simulink model "current_commutated_chopper"  (Simulink 7.5)
settings: Solver=ode45  StartTime=0.0  StopTime=.1  RelTol=1e-3
libraries: powerlib x13
settings Model: Creator=Smrit  LastModifiedBy=Sambhav
settings OptimizationCC: InitFltsAndDblsToZero=on
settings DebuggingCC: SaveWithParameterizedLinksMsg=none  StrictBusMsg=Warning

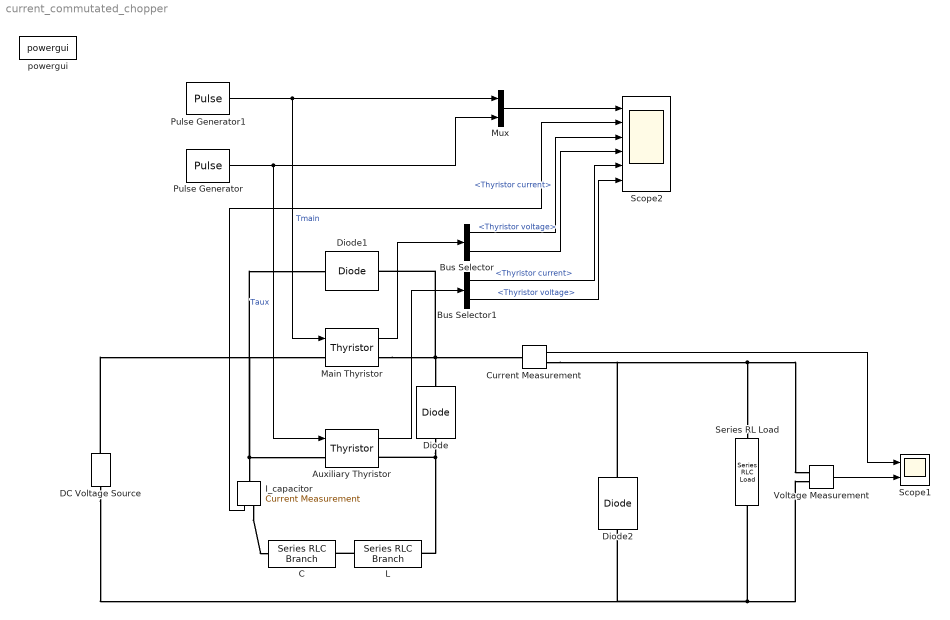
== system current_commutated_chopper ==
  Auxiliary Thyristor : powerlib/Power Electronics/Thyristor  DialogController=POWERSYS.PowerSysDialog  SystemSampleTime=-1  Ron=0.001  Lon=0  Vf=0.8  IC=0  Rs=500  Cs=250e-9  Measurements=on
  Bus Selector : BusSelector  OutputSignals=Thyristor current,Thyristor voltage
  Bus Selector1 : BusSelector  OutputSignals=Thyristor current,Thyristor voltage
  C : powerlib/Elements/Series RLC Branch  DialogController=POWERSYS.PowerSysDialog  PhysicalDomain=powersysdomain  SubClassName=unknown  LeftPortType=p1  RightPortType=p1  LConnTagsString=__new0  RConnTagsString=__new0  BranchType=C  Resistance=1  Inductance=1e-3  SetiL0=off  InitialCurrent=0  Capacitance=1e-6  Setx0=on  InitialVoltage=230  Measurements=None
  Current Measurement : powerlib/Measurements/Current Measurement  DialogController=POWERSYS.PowerSysDialog  SystemSampleTime=-1  PhasorSimulation=off  OutputType=Complex  PSBequivalent=0
  DC Voltage Source : powerlib/Electrical Sources/DC Voltage Source  DialogController=POWERSYS.PowerSysDialog  SystemSampleTime=-1  Amplitude=230  Measurements=None
  Diode : powerlib/Power Electronics/Diode  DialogController=POWERSYS.PowerSysDialog  SystemSampleTime=-1  Ron=0.001  Lon=0  Vf=0.8  IC=0  UseSnubber=off  Rs=500  Cs=250e-9  Measurements=off
  Diode1 : powerlib/Power Electronics/Diode  DialogController=POWERSYS.PowerSysDialog  SystemSampleTime=-1  Ron=0.001  Lon=0  Vf=0.8  IC=0  UseSnubber=off  Rs=500  Cs=250e-9  Measurements=off
  Diode2 : powerlib/Power Electronics/Diode  DialogController=POWERSYS.PowerSysDialog  SystemSampleTime=-1  Ron=0.001  Lon=0  Vf=0.8  IC=0  UseSnubber=off  Rs=500  Cs=250e-9  Measurements=off
  I_capacitor : powerlib/Measurements/Current Measurement  DialogController=POWERSYS.PowerSysDialog  SystemSampleTime=-1  PhasorSimulation=off  OutputType=Complex  PSBequivalent=0
  L : powerlib/Elements/Series RLC Branch  DialogController=POWERSYS.PowerSysDialog  PhysicalDomain=powersysdomain  SubClassName=unknown  LeftPortType=p1  RightPortType=p1  LConnTagsString=__new0  RConnTagsString=__new0  BranchType=L  Resistance=1  Inductance=1e-3  SetiL0=off  InitialCurrent=0  Capacitance=1e-6  Setx0=off  InitialVoltage=0  Measurements=None
  Main Thyristor : powerlib/Power Electronics/Thyristor  DialogController=POWERSYS.PowerSysDialog  SystemSampleTime=-1  Ron=0.001  Lon=0  Vf=0.8  IC=0  Rs=500  Cs=250e-9  Measurements=on
  Mux : Mux  Inputs=2
  Pulse Generator : DiscretePulseGenerator  PulseType=Time based  Amplitude=1  Period=20e-3  PulseWidth=.5  PhaseDelay=10e-3  SampleTime=1
  Pulse Generator1 : DiscretePulseGenerator  PulseType=Time based  Amplitude=1  Period=20e-3  PulseWidth=.5  PhaseDelay=5e-3  SampleTime=1
  Scope1 : Scope  NumInputPorts=2
      settings: YMin=-0.5~-0.2  YMax=3.5~300
  Scope2 : Scope  NumInputPorts=6
      settings: TimeRange=0.01606557841592294  YMin=0~-7~0~-10~0~-10  YMax=1.25~7~4~300~10~300  SaveName=ScopeData2
  Series RL Load : powerlib/Elements/Series RLC Load  DialogController=POWERSYS.PowerSysDialog  PhysicalDomain=powersysdomain  SubClassName=unknown  LeftPortType=p1  RightPortType=p1  LConnTagsString=a  RConnTagsString=__new0  NominalVoltage=1000  NominalFrequency=50  ActivePower=10e3  InductivePower=100  CapacitivePower=0  Setx0=off  InitialVoltage=0  SetiL0=off  InitialCurrent=0  Measurements=None
  Voltage Measurement : powerlib/Measurements/Voltage Measurement  DialogController=POWERSYS.PowerSysDialog  SystemSampleTime=-1  PhasorSimulation=off  OutputType=Complex  PSBequivalent=0
  powergui : powerlib/powergui  SystemSampleTime=-1  SimulationMode=Continuous  SampleTime=50e-6  frequency=60  SPID=off  DisableSnubberDevices=off  DisableRonSwitches=off  DisableVfSwitches=off  SwTol=0  Interpol=off  frequencyindice=0  echomessages=off  HookPort=off  DisplayEquations=off  FunctionMessages=off  EnableUseOfTLC=off  x0status=blocks  RestoreLinks=warning  ResistiveCurrentMeasurement=off  Frange=[0:2:500]  Ylog=off  Xlog=on  ShowGrid=off  save=off  variable=ZData  ZoomFFT=on  StartTime=0.0  cycles=1  DisplayStyle=1  fundamental=60  FreqAxis=off  MaxFrequency=1000  frequencyindicesteady=1  RmsSteady=1  display=off  Ts=0  methode=off
  wires:
  Pulse Generator1/1 -> Main Thyristor/1, Mux/1  "Tmain"
  Pulse Generator/1 -> Auxiliary Thyristor/1, Mux/2  "Taux"
  Current Measurement/1 -> Scope1/1
  Voltage Measurement/1 -> Scope1/2
  Main Thyristor/1 -> Bus Selector/1
  Auxiliary Thyristor/1 -> Bus Selector1/1
  Bus Selector/1 -> Scope2/3  "<Thyristor current>"
  Bus Selector/2 -> Scope2/4  "<Thyristor voltage>"
  Bus Selector1/1 -> Scope2/5  "<Thyristor current>"
  Bus Selector1/2 -> Scope2/6  "<Thyristor voltage>"
  Mux/1 -> Scope2/1
  I_capacitor/1 -> Scope2/2
  connections:
  Main Thyristor/RConn1 -- Current Measurement/LConn1 -- Diode1/LConn1 -- Diode/RConn1
  Current Measurement/RConn1 -- Diode2/RConn1 -- Series RL Load/LConn1 -- Voltage Measurement/LConn1
  DC Voltage Source/LConn1 -- Diode2/LConn1 -- Series RL Load/RConn1 -- Voltage Measurement/LConn2
  Diode/LConn1 -- Auxiliary Thyristor/RConn1 -- L/RConn1
  L/LConn1 -- C/RConn1
  I_capacitor/RConn1 -- C/LConn1
  DC Voltage Source/RConn1 -- Diode1/RConn1 -- Main Thyristor/LConn1 -- I_capacitor/LConn1 -- Auxiliary Thyristor/LConn1
